simulink model "vehicle_detection"  (R2023a)
settings: Solver=VariableStepAuto  StartTime=0.0  StopTime=10.0  RelTol=1e-3
libraries: visionconversions x1, visionsources x1, visionanalysis x1
settings Model: Creator=spandhansrirag  LastModifiedBy=spandhansrirag

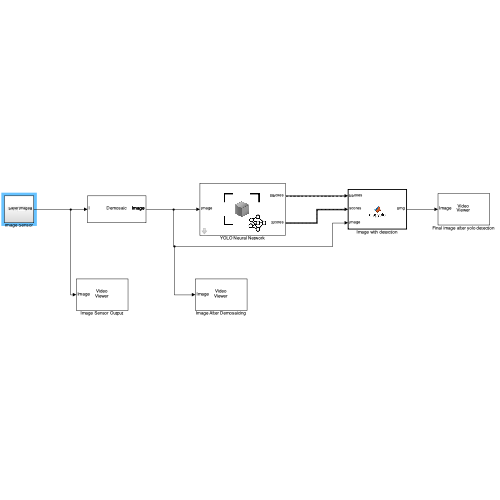
[thumbnail: Simulink's stored preview of the top-level diagram]
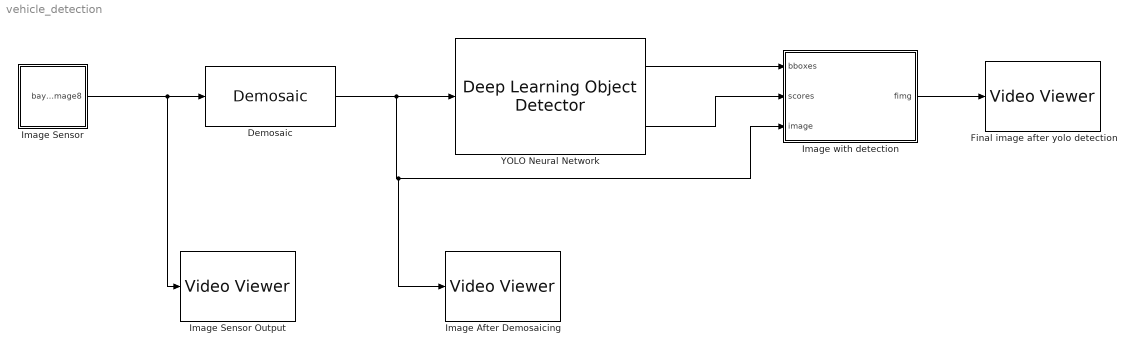
== system vehicle_detection ==
  Demosaic : visionconversions/Demosaic  algorithm=Obsolete  algorithmActive=Bilinear  alignment=RGGB  imagePorts=One multidimensional signal  roundingMode=Floor  overflowMode=on  prodOutputMode=Binary point scaling  prodOutputWordLength=32  prodOutputFracLength=10
  Final image after yolo detection : VideoViewer  FigPos=[547 683 380 259]
  Image After Demosaicing : VideoViewer  FigPos=[527 755 418 304]
  Image Sensor : Subsystem
  Image Sensor Output : VideoViewer  FigPos=[804 675 418 304]
  Image with detection : MATLAB Function  TreatAsAtomicUnit=on
  YOLO Neural Network : visionanalysis/Deep Learning Object Detector  Detector=Detector from MAT-file  DetectorFunction=untitled  DetectorFilePath=/Users/spandhansrirag/Documents/MATLAB/Examples/R2023a/deeplearning_shared/ObjectDetectionUsingYOLOV2DeepLearningExample/yolotrained_data.mat  MaxDetections=10  Bboxes=on  Scores=on  UseROI=off  ROI=[1 1 100 100]  Threshold=0.3  NumStrongestRegions=2000  UseMinSize=off  MinSize=[1 1]  UseMaxSize=off  MaxSize=[50 50]  ForceInterpretedSim=off
  wires:
  YOLO Neural Network/2 -> Image with detection/2(scores)
  YOLO Neural Network/1 -> Image with detection/1(bboxes)
  Image with detection/1(fimg) -> Final image after yolo detection/1
  Demosaic/1 -> Image After Demosaicing/1, Image with detection/3(image), YOLO Neural Network/1
  Image Sensor/1(bayerImage8) -> Image Sensor Output/1, Demosaic/1

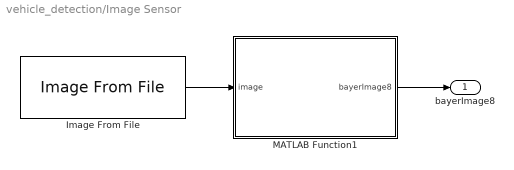
== system vehicle_detection/Image Sensor ==
  Image From File : visionsources/Image From File  Tag=vipblks_nd  FileName=/Users/spandhansrirag/Documents/MATLAB/Examples/R2023a/deeplearning_shared/ObjectDetectionUsingYOLOV2DeepLearningExample/vehicleImages/image_00007.jpg  Ts=1  imagePorts=One multidimensional signal  OutPortLabels=R|G|B  ImageDataType=Inherit from input image  sdImageDataType=uint(8)  Signed=on  WordLength=16  FractionLengthMode=User-defined  FractionLength=15
  MATLAB Function1 : MATLAB Function  TreatAsAtomicUnit=on
  bayerImage8 : Outport
  wires:
  MATLAB Function1/1(bayerImage8) -> bayerImage8/1
  Image From File/1 -> MATLAB Function1/1(image)

== matlab function vehicle_detection/Image Sensor/MATLAB Function1 ==
  data: image input; bayerImage8 output
function bayerImage8 = Mosaic(image)
%function bayerff8 = Mosaic(image)
img = image;
%imshow(img) 
[rows, cols, depth] = size(img);

% Create empty matrices for the Bayer channels
redChannel = zeros(rows, cols);
greenChannel = zeros(rows, cols);
blueChannel = zeros(rows, cols);

% Assign the RGB values to Bayer channels based on the Bayer pattern (e.g., RGGB)
for i = 1:rows
    for j = 1:cols
        if mod(i, 2) == 1 % Odd rows
            if mod(j, 2) == 1 % Odd columns
                redChannel(i, j) = img(i, j, 1); % Red pixel
            else
                greenChannel(i, j) = img(i, j, 2); % Green pixel
            end
        else % Even rows
            if mod(j, 2) == 1 % Odd columns
                greenChannel(i, j) = img(i, j, 2); % Green pixel
            else
                blueChannel(i, j) = img(i, j, 3); % Blue pixel
            end
        end
    end
end
redChannel8 = uint8(redChannel);
blueChannel8 = uint8(blueChannel);
greenChannel8 = uint8(greenChannel);
%bayerImage in double
bayerImage = redChannel + greenChannel + blueChannel; 
%bayerImage in uint8
bayerImage8 = redChannel8 + greenChannel8 + blueChannel8;
%imshow(bayerImage8)
reconsImage8 = demosaic(bayerImage8,"rggb");
%imshow(reconsImage8)
bayerff8=cat(3,redChannel8,greenChannel8,blueChannel8);
%end

== matlab function vehicle_detection/Image with detection ==
  data: bboxes input; fimg output; scores input; image input
function fimg = dispyolo(bboxes,scores,image)

fimg = insertObjectAnnotation(image,'rectangle',bboxes,scores);
